simulink library "issLVLHPointingSim_sl"  (R2024b)
settings: Solver=VariableStepAuto  StartTime=0.0  StopTime=10.0  RelTol=1e-3
undefined symbols (not defined in the file): adcsParams, hwParams, satDynParams
libraries: satAttDcmPDController_sl x1, atmoAttDisturbanceISS_sl x1, satEulerDyn_sl x1, satAttKinematics_sl x1, dgcmgFourParallelArray_sl x1, earthHorizonSensorHW_sl x1, gimbalSensorHW_sl x1, gyroSensorHW_sl x1, magnetometerSensorHW_sl x1
settings Model: Creator=gilbu
settings RTWCC: GPUComputeCapability=3.5

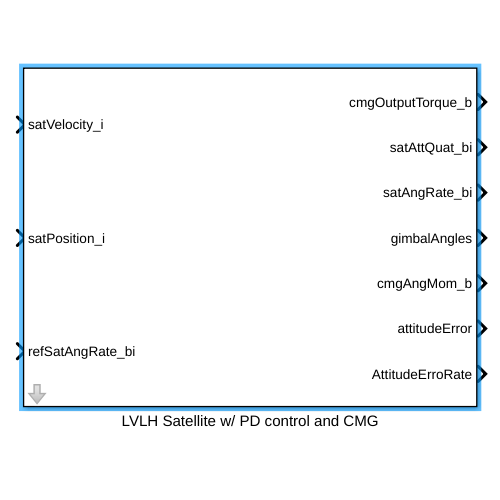
[thumbnail: Simulink's stored preview of the top-level diagram]
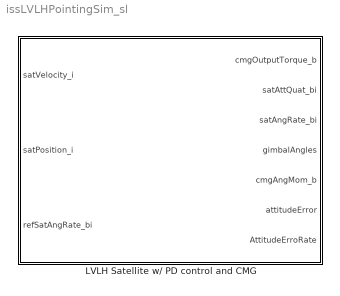
== system issLVLHPointingSim_sl ==
  LVLH Satellite w/ PD control and CMG : Subsystem  mask{adcsParams=adcsParams, hwParams=hwParams, satDynParams=satDynParams}
      mask prompts: adcsParams "ADCS Parameters <struct>"; hwParams "Hardware Parameters <struct>"; satDynParams "Satellite Dynamics and Kinematic parameters <struct>"
      mask DialogControl DescTextVar Prompt: Simulation of rigid body satellite in circular orbit. Use three reaction wheels, a ADCS based on DCM error and PD controller. Includes option to add sensor and actuator noise.Author: Antonio Gil Buitrago

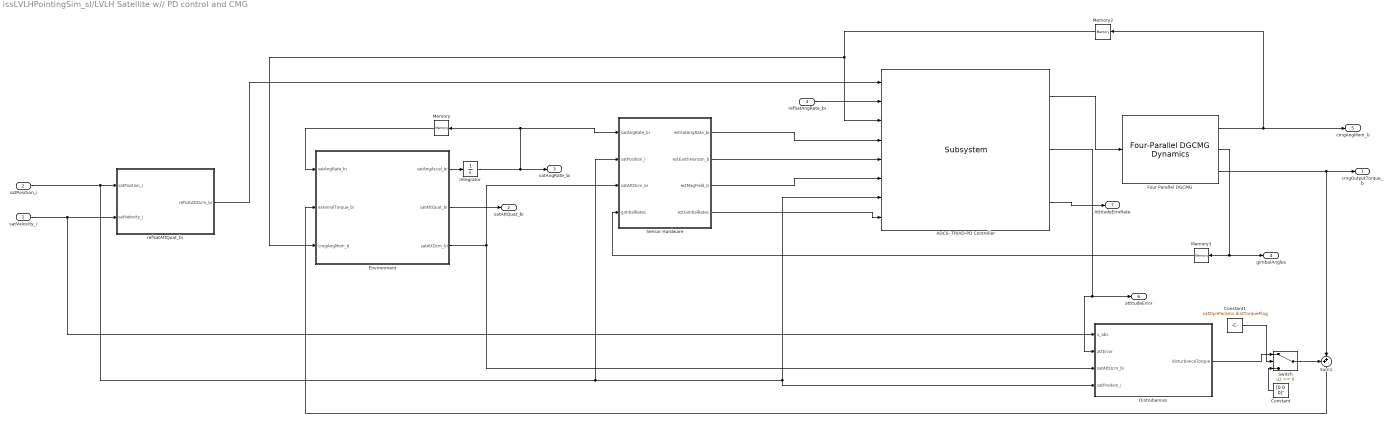
== system issLVLHPointingSim_sl/LVLH Satellite w// PD control and CMG ==
  satVelocity_i : Inport
  satPosition_i : Inport  Port=2
  refSatAngRate_bi : Inport  Port=3
  ADCS- TRIAD-PD Controller : satAttDcmPDController_sl/Subsystem  kP=adcsParams.kP  kD=adcsParams.kD  rotorInertia=hwParams.rotorInertia  rotorAngRate=hwParams.rotorAngRate  maxGimbalRate=hwParams.maxGimbalRate  innerAngDistGain=adcsParams.innerAngDistGain  outerAngDistGain=adcsParams.outerAngDistGain  satInertiaTensor=satDynParams.satInertiaTensor
      link override Max Gimbal Rates: UpperLimit=hwParams.maxGimbalRates  LowerLimit=-hwParams.maxGimbalRates
  Constant : Constant  Value=[0 0 0]'
  Constant1 : Constant  Value=satDynParams.distTorqueFlag
  Distrubances : Subsystem
  Environment : Subsystem
  Four Parallel DGCMG : dgcmgFourParallelArray_sl/Four-Parallel DGCMG Dynamics  rotorInertia=hwParams.rotorInertia  rotorAngRate=hwParams.rotorAngRate  Parameter3=hwParams.gimbalAngRates0
      link override Integrator: InitialCondition=hwParams.gimbalAngRates0
  Integrator : Integrator  InitialCondition=satDynParams.satAngRate0
  Memory : Memory  InitialCondition=satDynParams.satAngRate0
  Memory2 : Memory  InitialCondition=[0 0 0]'
  Memory3 : Memory  InitialCondition=hwParams.gimbalAngles0
  Sensor Hardware : Subsystem
  Sum1 : Sum  Inputs=++|
  Switch : Switch  SaturateOnIntegerOverflow=off  InputSameDT=off
  refSatAttQuat_bi : MATLAB Function  TreatAsAtomicUnit=on
  cmgOutputTorque_b : Outport
  satAttQuat_bi : Outport  Port=2
  satAngRate_bi : Outport  Port=3
  gimbalAngles : Outport  Port=4
  cmgAngMom_b : Outport  Port=5
  attitudeError : Outport  Port=6
  AttitudeErroRate : Outport  Port=7
  wires:
  refSatAngRate_bi/1 -> ADCS- TRIAD-PD Controller/2
  refSatAttQuat_bi/1(refSatAttDcm_bi) -> ADCS- TRIAD-PD Controller/1
  Integrator/1 -> Memory/1, Sensor Hardware/1(satAngRate_bi), satAngRate_bi/1
  satPosition_i/1 -> Distrubances/4(satPosition_i), ADCS- TRIAD-PD Controller/7, Sensor Hardware/2(satPosition_i), refSatAttQuat_bi/1(satPosition_i)
  Environment/3(satAttDcm_bi) -> Distrubances/3(satAttDcm_bi), Sensor Hardware/3(satAttDcm_bi)
  Sensor Hardware/2(estEarthHorizon_b) -> ADCS- TRIAD-PD Controller/5
  Sensor Hardware/3(estMagField_b) -> ADCS- TRIAD-PD Controller/6
  Environment/1(satAngAccel_bi) -> Integrator/1
  Environment/2(satAttQuat_bi) -> satAttQuat_bi/1
  satVelocity_i/1 -> Distrubances/1(v_abs), refSatAttQuat_bi/2(satVelocity_i)
  Four Parallel DGCMG/3 -> Sum1/2, cmgOutputTorque_b/1
  Four Parallel DGCMG/1 -> Memory2/1, cmgAngMom_b/1
  Memory2/1 -> Environment/3(cmgAngMom_b), ADCS- TRIAD-PD Controller/3
  ADCS- TRIAD-PD Controller/1 -> Four Parallel DGCMG/1
  Four Parallel DGCMG/2 -> gimbalAngles/1, Memory3/1
  Sum1/1 -> Environment/2(externalTorque_bi)
  Memory/1 -> Environment/1(satAngRate_bi)
  Sensor Hardware/1(estSatAngRate_bi) -> ADCS- TRIAD-PD Controller/4
  Memory3/1 -> Sensor Hardware/4(gimbalRates)
  Sensor Hardware/4(estGimbalRates) -> ADCS- TRIAD-PD Controller/8
  ADCS- TRIAD-PD Controller/2 -> attitudeError/1, Distrubances/2(attError)
  ADCS- TRIAD-PD Controller/3 -> AttitudeErroRate/1
  Switch/1 -> Sum1/1
  Distrubances/1(disturbanceTorque) -> Switch/1
  Constant/1 -> Switch/3
  Constant1/1 -> Switch/2

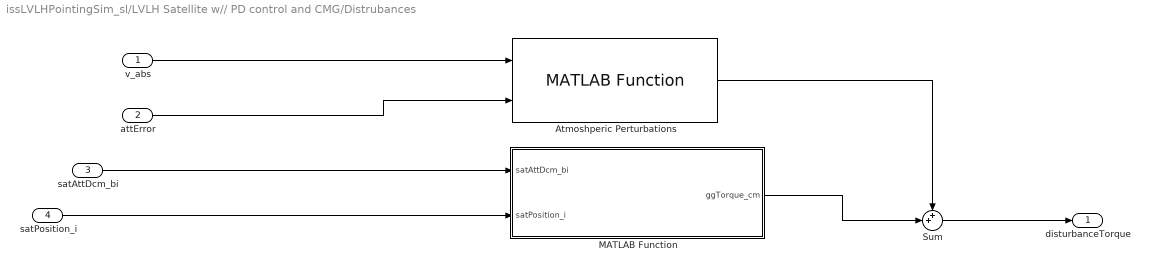
== system issLVLHPointingSim_sl/LVLH Satellite w// PD control and CMG/Distrubances ==
  v_abs : Inport
  attError : Inport  Port=2
  satAttDcm_bi : Inport  Port=3
  satPosition_i : Inport  Port=4
  Atmoshperic Perturbations : atmoAttDisturbanceISS_sl/MATLAB Function
  MATLAB Function : MATLAB Function  TreatAsAtomicUnit=on
  Sum : Sum  Inputs=++|
  disturbanceTorque : Outport
  wires:
  Sum/1 -> disturbanceTorque/1
  MATLAB Function/1(ggTorque_cm) -> Sum/2
  satAttDcm_bi/1 -> MATLAB Function/1(satAttDcm_bi)
  Atmoshperic Perturbations/1 -> Sum/1
  v_abs/1 -> Atmoshperic Perturbations/1
  attError/1 -> Atmoshperic Perturbations/2
  satPosition_i/1 -> MATLAB Function/2(satPosition_i)

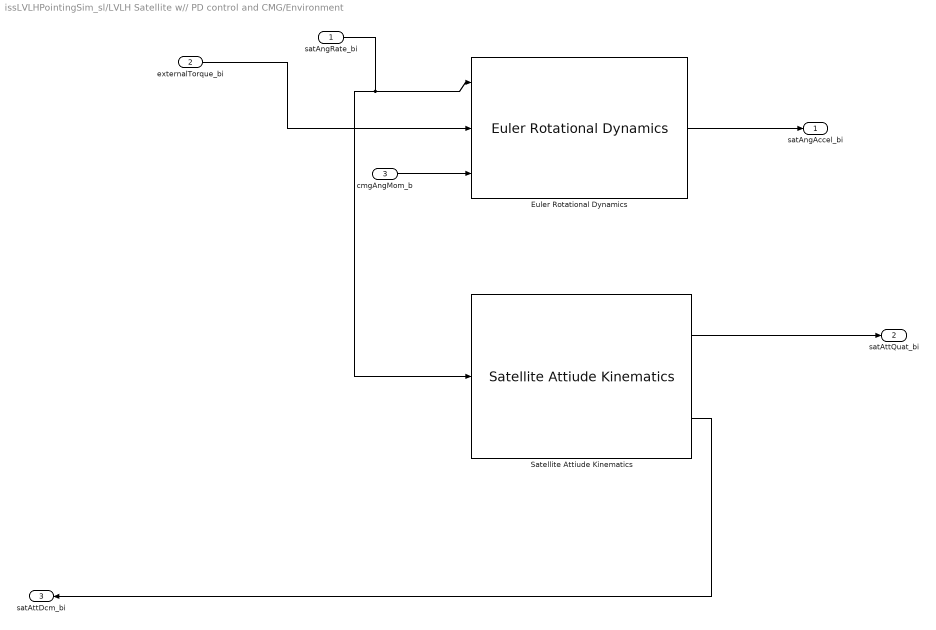
== system issLVLHPointingSim_sl/LVLH Satellite w// PD control and CMG/Environment ==
  satAngRate_bi : Inport
  externalTorque_bi : Inport  Port=2
  cmgAngMom_b : Inport  Port=3
  "Euler Rotational Dynamics " : satEulerDyn_sl/Euler Rotational Dynamics   satInertiaTensor=satDynParams.satInertiaTensor
  Satellite Attiude Kinematics : satAttKinematics_sl/Satellite Attiude Kinematics  satAttQuat0=satDynParams.satAttQuat0  satAttDcm0=satDynParams.satAttDcm0
  satAngAccel_bi : Outport
  satAttQuat_bi : Outport  Port=2
  satAttDcm_bi : Outport  Port=3
  wires:
  satAngRate_bi/1 -> Satellite Attiude Kinematics/1, "Euler Rotational Dynamics "/1
  Satellite Attiude Kinematics/1 -> satAttQuat_bi/1
  "Euler Rotational Dynamics "/1 -> satAngAccel_bi/1
  Satellite Attiude Kinematics/2 -> satAttDcm_bi/1
  externalTorque_bi/1 -> "Euler Rotational Dynamics "/2
  cmgAngMom_b/1 -> "Euler Rotational Dynamics "/3

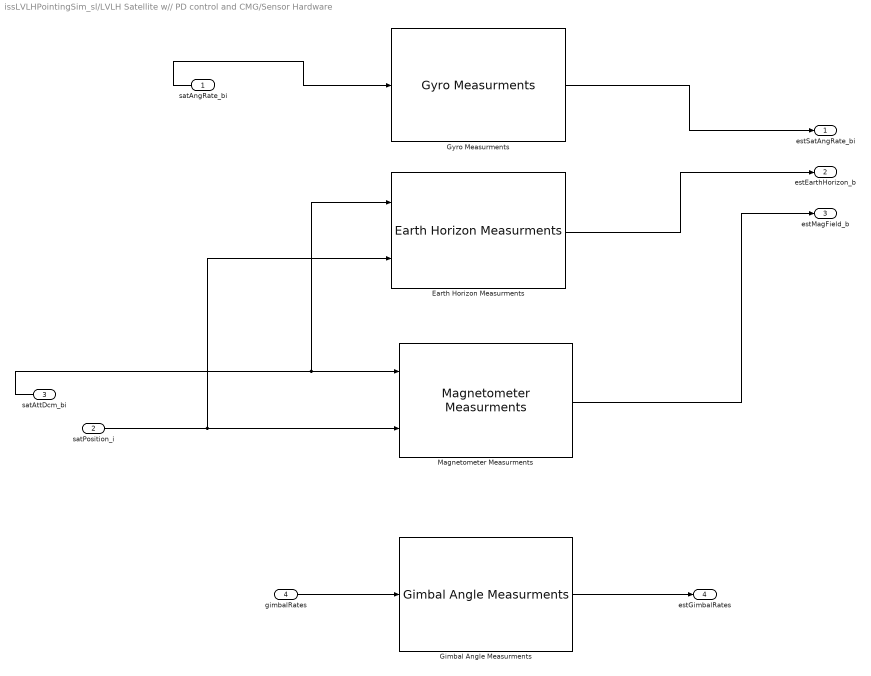
== system issLVLHPointingSim_sl/LVLH Satellite w// PD control and CMG/Sensor Hardware ==
  satAngRate_bi : Inport
  satPosition_i : Inport  Port=2
  satAttDcm_bi : Inport  Port=3
  gimbalRates : Inport  Port=4
  Earth Horizon Measurments : earthHorizonSensorHW_sl/Earth Horizon Measurments  earthHorizonErrorFlag=hwParams.earthHorizonErrorFlag  earthHorizonErrorDcm=hwParams.earthHorizonErrorDcm
  Gimbal Angle Measurments : gimbalSensorHW_sl/Gimbal Angle Measurments  gimbalErrorFlag=hwParams.gimbalErrorFlag  gimbalBias=hwParams.gimbalBias  gimbalNoisePower=hwParams.gimbalNoisePower
  Gyro Measurments : gyroSensorHW_sl/Gyro Measurments  gyroErrorFlag=hwParams.gyroErrorFlag  gyroBias=hwParams.gyroBias  gyroNoisePower=hwParams.gyroNoisePower
  Magnetometer Measurments : magnetometerSensorHW_sl/Magnetometer Measurments  magErrorFlag=hwParams.magErrorFlag  magError=hwParams.magError
  estSatAngRate_bi : Outport
  estEarthHorizon_b : Outport  Port=2
  estMagField_b : Outport  Port=3
  estGimbalRates : Outport  Port=4
  wires:
  satPosition_i/1 -> Earth Horizon Measurments/2, Magnetometer Measurments/2
  Magnetometer Measurments/1 -> estMagField_b/1
  satAngRate_bi/1 -> Gyro Measurments/1
  Gyro Measurments/1 -> estSatAngRate_bi/1
  satAttDcm_bi/1 -> Earth Horizon Measurments/1, Magnetometer Measurments/1
  Earth Horizon Measurments/1 -> estEarthHorizon_b/1
  gimbalRates/1 -> Gimbal Angle Measurments/1
  Gimbal Angle Measurments/1 -> estGimbalRates/1

== matlab function issLVLHPointingSim_sl/LVLH Satellite w// PD control and CMG/refSatAttQuat_bi ==
  data: refSatAttDcm_bi output; satPosition_i input; satVelocity_i input
function refSatAttDcm_bi = refAttDcm ( ...
    satPosition_i,satVelocity_i)
%----------------------------------------------------------------------
% Calcualte Ref Sat Att DCM from inertial position and velocity
     rHat = satPosition_i./norm(satPosition_i);
    vHat = satVelocity_i./norm(satVelocity_i);
    crossVec = cross(-rHat,vHat);
    yHat = crossVec./norm(crossVec);
    refSatAttDcm_bi= [vHat'; yHat'; -rHat'];
  
end

== matlab function issLVLHPointingSim_sl/LVLH Satellite w// PD control and CMG/Distrubances/MATLAB Function ==
  data: ggTorque_cm output; satAttDcm_bi input size=3,3; satPosition_i input size=3
function ggTorque_cm = gravity_gradient ( ...
    satAttDcm_bi,satPosition_i)...%inputs)
%-------------------------------------------------------------------------------
%Torque Calculations

r_b= satAttDcm_bi*satPosition_i; % [m]
mu = 3.98e14; %m^3/s^2

Jb = [70942261    0 0; 0  59070966   0; 0   0 123909888];
      %  [70942261 3512761 3543989;
      % 3512761 59070966 -2768801;   %kg*m^2
      % 3543989 -2768801 123909888];

nr = norm (r_b);
db= -r_b/nr;

ggTorque_cm = 3*mu/nr^3*cross(db, Jb*db); %N*m
